simulink model "closed_loop_plant"  (R2018b)
settings: Solver=VariableStepAuto  StartTime=0.0  StopTime=10.0  RelTol=1e-3
settings Model: Creator=kletech  LastModifiedBy=kletech

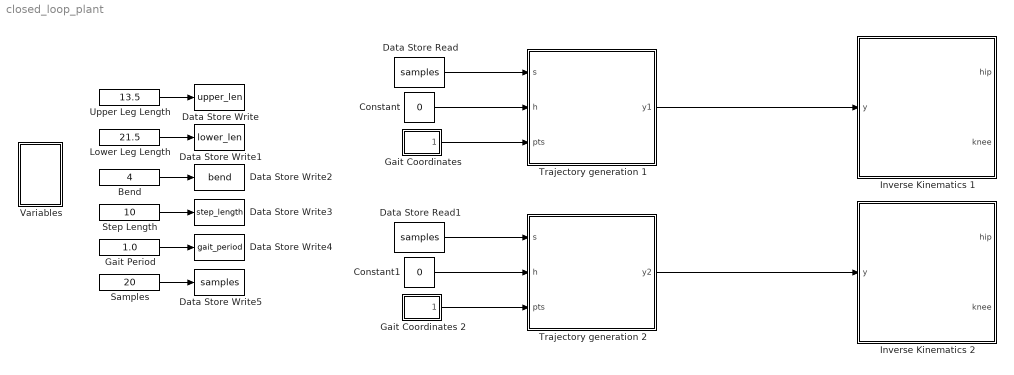
== system closed_loop_plant ==
  "Bend " : Constant  Value=4
  Constant : Constant  Value=0
  Constant1 : Constant  Value=0
  Data Store Read : DataStoreRead  DataStoreName=samples
  Data Store Read1 : DataStoreRead  DataStoreName=samples
  Data Store Write : DataStoreWrite  DataStoreName=upper_len
  Data Store Write1 : DataStoreWrite  DataStoreName=lower_len
  Data Store Write2 : DataStoreWrite  DataStoreName=bend
  Data Store Write3 : DataStoreWrite  DataStoreName=step_length
  Data Store Write4 : DataStoreWrite  DataStoreName=gait_period
  Data Store Write5 : DataStoreWrite  DataStoreName=samples
  Gait Coordinates : Subsystem
  Gait Coordinates 2 : Subsystem
  Gait Period : Constant  Value=1.0
  Inverse Kinematics 1 : Subsystem
  Inverse Kinematics 2 : Subsystem
  Lower Leg Length : Constant  Value=21.5
  Samples : Constant  Value=20
  Step Length : Constant  Value=10
  Trajectory generation 1 : Subsystem
  Trajectory generation 2 : Subsystem
  "Upper Leg Length " : Constant  Value=13.5
  "Variables " : Subsystem
  wires:
  Gait Period/1 -> Data Store Write4/1
  "Bend "/1 -> Data Store Write2/1
  "Upper Leg Length "/1 -> Data Store Write/1
  Lower Leg Length/1 -> Data Store Write1/1
  Step Length/1 -> Data Store Write3/1
  Samples/1 -> Data Store Write5/1
  Gait Coordinates/1(Out1) -> Trajectory generation 1/3(pts)
  Constant/1 -> Trajectory generation 1/2(h)
  Data Store Read/1 -> Trajectory generation 1/1("s ")
  Constant1/1 -> Trajectory generation 2/2(h)
  Gait Coordinates 2/1(Out1) -> Trajectory generation 2/3(pts)
  Data Store Read1/1 -> Trajectory generation 2/1("s ")
  Trajectory generation 1/1(y1) -> Inverse Kinematics 1/1(y)
  Trajectory generation 2/1(y2) -> Inverse Kinematics 2/1(y)

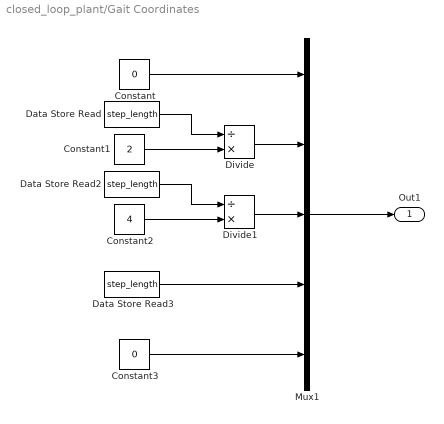
== system closed_loop_plant/Gait Coordinates ==
  Constant : Constant  Value=0
  Constant1 : Constant  Value=2
  Constant2 : Constant  Value=4
  Constant3 : Constant  Value=0
  Data Store Read : DataStoreRead  DataStoreName=step_length
  Data Store Read2 : DataStoreRead  DataStoreName=step_length
  Data Store Read3 : DataStoreRead  DataStoreName=step_length
  Divide : Product  Inputs=/*
  Divide1 : Product  Inputs=/*
  Mux1 : Mux  Inputs=5
  Out1 : Outport
  wires:
  Mux1/1 -> Out1/1
  Constant/1 -> Mux1/1
  Data Store Read/1 -> Divide/1
  Constant1/1 -> Divide/2
  Data Store Read2/1 -> Divide1/1
  Constant2/1 -> Divide1/2
  Divide/1 -> Mux1/2
  Divide1/1 -> Mux1/3
  Data Store Read3/1 -> Mux1/4
  Constant3/1 -> Mux1/5

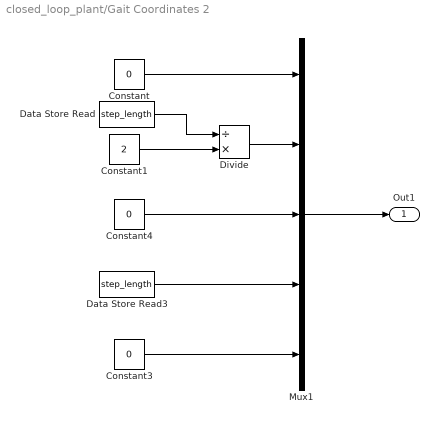
== system closed_loop_plant/Gait Coordinates 2 ==
  Constant : Constant  Value=0
  Constant1 : Constant  Value=2
  Constant3 : Constant  Value=0
  Constant4 : Constant  Value=0
  Data Store Read : DataStoreRead  DataStoreName=step_length
  Data Store Read3 : DataStoreRead  DataStoreName=step_length
  Divide : Product  Inputs=/*
  Mux1 : Mux  Inputs=5
  Out1 : Outport
  wires:
  Mux1/1 -> Out1/1
  Constant/1 -> Mux1/1
  Data Store Read/1 -> Divide/1
  Constant1/1 -> Divide/2
  Divide/1 -> Mux1/2
  Data Store Read3/1 -> Mux1/4
  Constant3/1 -> Mux1/5
  Constant4/1 -> Mux1/3

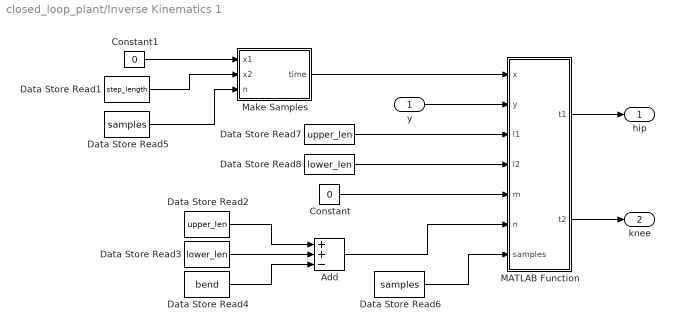
== system closed_loop_plant/Inverse Kinematics 1 ==
  y : Inport
  Add : Sum  Inputs=++-
  Constant : Constant  Value=0
  Constant1 : Constant  Value=0
  Data Store Read1 : DataStoreRead  DataStoreName=step_length
  Data Store Read2 : DataStoreRead  DataStoreName=upper_len
  Data Store Read3 : DataStoreRead  DataStoreName=lower_len
  Data Store Read4 : DataStoreRead  DataStoreName=bend
  Data Store Read5 : DataStoreRead  DataStoreName=samples
  Data Store Read6 : DataStoreRead  DataStoreName=samples
  Data Store Read7 : DataStoreRead  DataStoreName=upper_len
  Data Store Read8 : DataStoreRead  DataStoreName=lower_len
  MATLAB Function : MATLAB Function  TreatAsAtomicUnit=on
  "Make Samples " : MATLAB Function  TreatAsAtomicUnit=on
  hip : Outport
  knee : Outport  Port=2
  wires:
  MATLAB Function/1(t1) -> hip/1
  MATLAB Function/2(t2) -> knee/1
  Data Store Read3/1 -> Add/2
  Data Store Read2/1 -> Add/1
  Data Store Read4/1 -> Add/3
  Add/1 -> MATLAB Function/6(n)
  Constant/1 -> MATLAB Function/5(m)
  y/1 -> MATLAB Function/2(y)
  Constant1/1 -> "Make Samples "/1(x1)
  Data Store Read1/1 -> "Make Samples "/2(x2)
  Data Store Read6/1 -> MATLAB Function/7(samples)
  Data Store Read5/1 -> "Make Samples "/3(n)
  "Make Samples "/1(time) -> MATLAB Function/1(x)
  Data Store Read8/1 -> MATLAB Function/4(l2)
  Data Store Read7/1 -> MATLAB Function/3(l1)

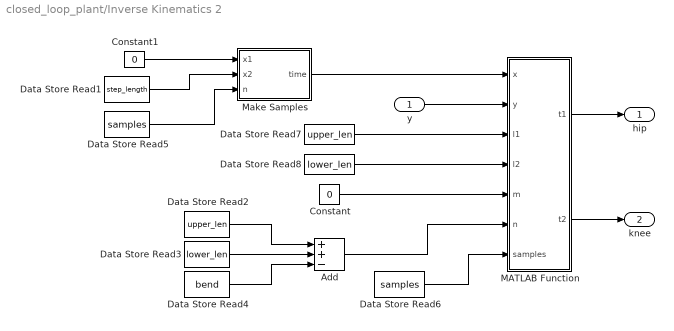
== system closed_loop_plant/Inverse Kinematics 2 ==
  y : Inport
  Add : Sum  Inputs=++-
  Constant : Constant  Value=0
  Constant1 : Constant  Value=0
  Data Store Read1 : DataStoreRead  DataStoreName=step_length
  Data Store Read2 : DataStoreRead  DataStoreName=upper_len
  Data Store Read3 : DataStoreRead  DataStoreName=lower_len
  Data Store Read4 : DataStoreRead  DataStoreName=bend
  Data Store Read5 : DataStoreRead  DataStoreName=samples
  Data Store Read6 : DataStoreRead  DataStoreName=samples
  Data Store Read7 : DataStoreRead  DataStoreName=upper_len
  Data Store Read8 : DataStoreRead  DataStoreName=lower_len
  MATLAB Function : MATLAB Function  TreatAsAtomicUnit=on
  "Make Samples " : MATLAB Function  TreatAsAtomicUnit=on
  hip : Outport
  knee : Outport  Port=2
  wires:
  MATLAB Function/1(t1) -> hip/1
  MATLAB Function/2(t2) -> knee/1
  Data Store Read3/1 -> Add/2
  Data Store Read2/1 -> Add/1
  Data Store Read4/1 -> Add/3
  Add/1 -> MATLAB Function/6(n)
  Constant/1 -> MATLAB Function/5(m)
  y/1 -> MATLAB Function/2(y)
  Constant1/1 -> "Make Samples "/1(x1)
  Data Store Read1/1 -> "Make Samples "/2(x2)
  Data Store Read6/1 -> MATLAB Function/7(samples)
  Data Store Read5/1 -> "Make Samples "/3(n)
  "Make Samples "/1(time) -> MATLAB Function/1(x)
  Data Store Read8/1 -> MATLAB Function/4(l2)
  Data Store Read7/1 -> MATLAB Function/3(l1)

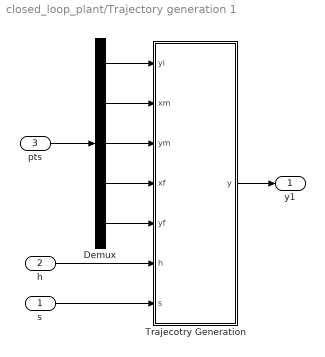
== system closed_loop_plant/Trajectory generation 1 ==
  "s " : Inport
  h : Inport  Port=2
  pts : Inport  Port=3
  Demux : Demux  Outputs=5
  Trajecotry Generation : MATLAB Function  TreatAsAtomicUnit=on
  y1 : Outport
  wires:
  Demux/2 -> Trajecotry Generation/2(xm)
  Demux/5 -> Trajecotry Generation/5(yf)
  Demux/3 -> Trajecotry Generation/3(ym)
  Demux/1 -> Trajecotry Generation/1(yi)
  pts/1 -> Demux/1
  Demux/4 -> Trajecotry Generation/4(xf)
  Trajecotry Generation/1(y) -> y1/1
  h/1 -> Trajecotry Generation/6(h)
  "s "/1 -> Trajecotry Generation/7(s)

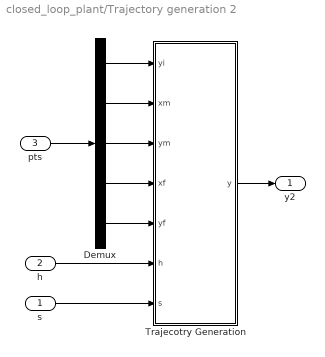
== system closed_loop_plant/Trajectory generation 2 ==
  "s " : Inport
  h : Inport  Port=2
  pts : Inport  Port=3
  Demux : Demux  Outputs=5
  Trajecotry Generation : MATLAB Function  TreatAsAtomicUnit=on
  y2 : Outport
  wires:
  Demux/2 -> Trajecotry Generation/2(xm)
  Demux/5 -> Trajecotry Generation/5(yf)
  Demux/3 -> Trajecotry Generation/3(ym)
  Demux/1 -> Trajecotry Generation/1(yi)
  pts/1 -> Demux/1
  Demux/4 -> Trajecotry Generation/4(xf)
  Trajecotry Generation/1(y) -> y2/1
  h/1 -> Trajecotry Generation/6(h)
  "s "/1 -> Trajecotry Generation/7(s)

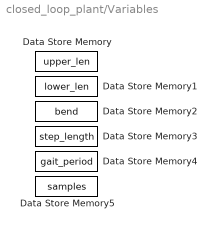
== system closed_loop_plant/Variables  ==
  Data Store Memory : DataStoreMemory  DataStoreName=upper_len  ReadBeforeWriteMsg=warning  WriteAfterWriteMsg=warning  WriteAfterReadMsg=warning  InitialValue=13.5  ShowAdditionalParam=off
  Data Store Memory1 : DataStoreMemory  DataStoreName=lower_len  ReadBeforeWriteMsg=warning  WriteAfterWriteMsg=warning  WriteAfterReadMsg=warning  InitialValue=21.5  ShowAdditionalParam=off
  Data Store Memory2 : DataStoreMemory  DataStoreName=bend  ReadBeforeWriteMsg=warning  WriteAfterWriteMsg=warning  WriteAfterReadMsg=warning  InitialValue=4  ShowAdditionalParam=off
  Data Store Memory3 : DataStoreMemory  DataStoreName=step_length  ReadBeforeWriteMsg=warning  WriteAfterWriteMsg=warning  WriteAfterReadMsg=warning  InitialValue=10  ShowAdditionalParam=off
  Data Store Memory4 : DataStoreMemory  DataStoreName=gait_period  ReadBeforeWriteMsg=warning  WriteAfterWriteMsg=warning  WriteAfterReadMsg=warning  InitialValue=1.0  ShowAdditionalParam=off
  Data Store Memory5 : DataStoreMemory  DataStoreName=samples  ReadBeforeWriteMsg=warning  WriteAfterWriteMsg=warning  WriteAfterReadMsg=warning  InitialValue=20  ShowAdditionalParam=off

== matlab function closed_loop_plant/Trajectory generation 1/Trajecotry Generation ==
  data: yi input; y output; xm input; ym input; xf input; yf input; h input; s input
function y = fcn(yi, xm,ym, xf,yf, h,s)
syms a b c;
eqn1 = c == yi;
eqn2 = ym == ((xm^2)*a + (xm*b) + c);
eqn3 = yf == ((xf^2)*a + (xf*b) + c);
[A,B] = equationsToMatrix([eqn1, eqn2, eqn3], [c, b, a]);
co_effs = linsolve(A,B);
x = linspace(h, h+xf, s);
y = double((co_effs(3)*((x-h).^2)) + (co_effs(2)*(x-h)) + co_effs(1));

== matlab function closed_loop_plant/Inverse Kinematics 1/Make Samples  ==
  data: x1 input; time output; x2 input; n input
function time = fcn(x1, x2, n)

time = linspace(x1, x2, n);

== matlab function closed_loop_plant/Trajectory generation 2/Trajecotry Generation ==
  data: yi input; y output; xm input; ym input; xf input; yf input; h input; s input
function y = fcn(yi, xm,ym, xf,yf, h,s)
syms a b c;
eqn1 = c == yi;
eqn2 = ym == ((xm^2)*a + (xm*b) + c);
eqn3 = yf == ((xf^2)*a + (xf*b) + c);
[A,B] = equationsToMatrix([eqn1, eqn2, eqn3], [c, b, a]);
co_effs = linsolve(A,B);
x = linspace(h, h+xf, s);
y = double((co_effs(3)*((x-h).^2)) + (co_effs(2)*(x-h)) + co_effs(1));

== matlab function closed_loop_plant/Inverse Kinematics 1/MATLAB Function ==
  data: x input; t1 output; y input; l1 input; l2 input; m input; n input; samples input; t2 output
function [t1, t2] = fcn(x, y, l1, l2, m, n, samples)
t2_numerator = ((x-m).^2 + (y-n).^2 - l1^2 - l2^2);
t2_denominator = (2 * l1 * l2);
t2 = acosd(t2_numerator./t2_denominator);

t1_numerator = l2 * sind(t2);
t1_denominator = l1 + (l2 * cosd(t2));
t1 = atand((y-n)./(x-m)) - atand(t1_numerator./t1_denominator);
t1((2*m) + 1 : samples) = t1((2*m) + 1 : samples) + 180;

t2 = -t2;
t1 = -180 -t1;

== matlab function closed_loop_plant/Inverse Kinematics 2/MATLAB Function ==
  data: x input; t1 output; y input; l1 input; l2 input; m input; n input; samples input; t2 output
function [t1, t2] = fcn(x, y, l1, l2, m, n, samples)
t2_numerator = ((x-m).^2 + (y-n).^2 - l1^2 - l2^2);
t2_denominator = (2 * l1 * l2);
t2 = acosd(t2_numerator./t2_denominator);

t1_numerator = l2 * sind(t2);
t1_denominator = l1 + (l2 * cosd(t2));
t1 = atand((y-n)./(x-m)) - atand(t1_numerator./t1_denominator);
t1((2*m) + 1 : samples) = t1((2*m) + 1 : samples) + 180;

t2 = -t2;
t1 = -180 -t1;

== matlab function closed_loop_plant/Inverse Kinematics 2/Make Samples  ==
  data: x1 input; time output; x2 input; n input
function time = fcn(x1, x2, n)

time = linspace(x1, x2, n);
